simulink library "RF_transformations"  (R2020b)
settings: Solver=VariableStepAuto  StartTime=0.0  StopTime=10.0  RelTol=1e-3
settings Model: Creator=matteolarcher  LastModifiedBy=matteolarcher

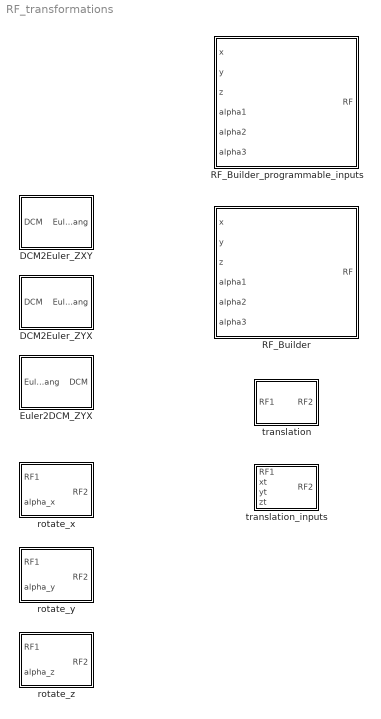
== system RF_transformations ==
  DCM2Euler_ZXY : MATLAB Function  TreatAsAtomicUnit=on
  DCM2Euler_ZYX : MATLAB Function  TreatAsAtomicUnit=on
  Euler2DCM_ZYX : MATLAB Function  TreatAsAtomicUnit=on
  RF_Builder : MATLAB Function  TreatAsAtomicUnit=on  mask{order_selector=['Z','Y','X']}
      mask prompts: order_selector "Rotation order"
      mask init:
      | switch order_selector
      |     case 1
      |         order = [1,2,3];
      |     case 2
      |         order = [1,3,2];
      |     case 3
      |         order = [2,1,3];
      |     case 4
      |         order = [2,3,1];
      |     case 5
      |         order = [3,2,1];
      |     case 6
      |         order = [3,1,2];
      |     case 7
      |         order = [1,2,1];
      |     case 8
      |         order = [1,3,1];
      |     case 9
      |         order = [2,1,2];
      |     case 10
      |         order = [2,3,2];
      |     case 11
      |         order = [3,1,3];
      |     case 12
      |         order = [3,2,3];
      | end
  RF_Builder_programmable_inputs : MATLAB Function  TreatAsAtomicUnit=on  mask{order_input=[3,2,1]}
      mask prompts: order_input "Rotation order"
      mask init:
      | % check input
      | if sum(order_input==1) ~= 1 || sum(order_input==2) ~= 1 || sum(order_input==3) ~= 1
      |     error("input must be provided in the format: [<axis1>,<axis2>,<axis3>], where axis can be 1 for X axis, 2 for Y axis or 3 fro Z axis");
      | end
      | 
      | order = order_input; 
      | 
      | % % assign rotation order
      | % order = [(1*(order_input(1)=='X'))+(2*(order_input(1)=='Y'))+(3*(order_input(1)=='Z')),...
      | %          (1*(order_input(2)=='X'))+(2*(order_input(2)=='Y'))+(3*(order_input(2)=='Z')),...
      | %          (1*(order_input(3)=='X'))+(2*(order_input(3)=='Y'))+(3*(order_input(3)=='Z'))];
  rotate_x : MATLAB Function  TreatAsAtomicUnit=on
  rotate_y : MATLAB Function  TreatAsAtomicUnit=on
  rotate_z : MATLAB Function  TreatAsAtomicUnit=on
  translation : MATLAB Function  TreatAsAtomicUnit=on  mask{xt=0, yt=0, zt=0}
      mask prompts: xt "x"; yt "y"; zt "z"
  translation_inputs : MATLAB Function  TreatAsAtomicUnit=on

== matlab function RF_transformations/DCM2Euler_ZYX ==
  data: DCM input; Euler_ang output
function Euler_ang  = fcn(DCM)

alpha_z = atan2(DCM(2,1),DCM(1,1));
alpha_y = -asin(DCM(3,1));
alpha_x = atan2(DCM(3,2),DCM(3,3));

Euler_ang = [alpha_z,alpha_y,alpha_x];

== matlab function RF_transformations/Euler2DCM_ZYX ==
  data: Euler_ang input; DCM output
function DCM  = fcn(Euler_ang)

alpha_z = Euler_ang(1);
alpha_y = Euler_ang(2);
alpha_x = Euler_ang(3);

DCM = [cos(alpha_z) * cos(alpha_y) -sin(alpha_z) * cos(alpha_x) + cos(alpha_z) * sin(alpha_y) * sin(alpha_x) sin(alpha_z) * sin(alpha_x) + cos(alpha_z) * sin(alpha_y) * cos(alpha_x); sin(alpha_z) * cos(alpha_y) cos(alpha_z) * cos(alpha_x) + sin(alpha_z) * sin(alpha_y) * sin(alpha_x) -cos(alpha_z) * sin(alpha_x) + sin(alpha_z) * sin(alpha_y) * cos(alpha_x); -sin(alpha_y) cos(alpha_y) * sin(alpha_x) cos(alpha_y) * cos(alpha_x)];

== matlab function RF_transformations/DCM2Euler_ZXY ==
  data: DCM input; Euler_ang output
function Euler_ang  = fcn(DCM)

alpha_x = asin(DCM(3,2));
alpha_y = -atan2(DCM(3,1),DCM(3,3));
alpha_z = -atan2(DCM(1,2),DCM(2,2));

Euler_ang = [alpha_z,alpha_x,alpha_y];

== matlab function RF_transformations/RF_Builder ==
  data: x input; RF output size=[4,4]; y input; z input; alpha1 input; alpha2 input; alpha3 input; order parameter
function RF = RF_Builder(x,y,z,alpha1,alpha2,alpha3,order)

RF = [1 0 0 x; 0 1 0 y; 0 0 1 z; 0 0 0 1;];

thetas = [alpha1,alpha2,alpha3];

for i = 1:3
    
    switch order(i)
        case 1
            theta = thetas(i);
            RX = [1 0 0 0; 0 cos(theta) -sin(theta) 0; 0 sin(theta) cos(theta) 0; 0 0 0 1;];
            RF = RF * RX;
        case 2
            theta = thetas(i);
            RY = [cos(theta) 0 sin(theta) 0; 0 1 0 0; -sin(theta) 0 cos(theta) 0; 0 0 0 1;];
            RF = RF * RY;
        case 3
            theta = thetas(i);
            RZ = [cos(theta) -sin(theta) 0 0; sin(theta) cos(theta) 0 0; 0 0 1 0; 0 0 0 1;];
            RF = RF * RZ;
    end
    
end

== matlab function RF_transformations/RF_Builder_programmable_inputs ==
  data: x input; RF output size=[4,4]; y input; z input; alpha1 input; alpha2 input; alpha3 input; order parameter
function RF = RF_Builder(x,y,z,alpha1,alpha2,alpha3,order)

RF = [1 0 0 x; 0 1 0 y; 0 0 1 z; 0 0 0 1;];

thetas = [alpha1,alpha2,alpha3];

for i = 1:3
    
    switch order(i)
        case 1
            theta = thetas(i);
            RX = [1 0 0 0; 0 cos(theta) -sin(theta) 0; 0 sin(theta) cos(theta) 0; 0 0 0 1;];
            RF = RF * RX;
        case 2
            theta = thetas(i);
            RY = [cos(theta) 0 sin(theta) 0; 0 1 0 0; -sin(theta) 0 cos(theta) 0; 0 0 0 1;];
            RF = RF * RY;
        case 3
            theta = thetas(i);
            RZ = [cos(theta) -sin(theta) 0 0; sin(theta) cos(theta) 0 0; 0 0 1 0; 0 0 0 1;];
            RF = RF * RZ;
    end
    
end

== matlab function RF_transformations/translation_inputs ==
  data: RF1 input size=[4,4]; RF2 output size=[4,4]; xt input; yt input; zt input
function RF2 = translation(RF1,xt, yt, zt)
RF2 = RF1*(eye(4) + [zeros(4,3) [xt,yt,zt,0]']);
end

== matlab function RF_transformations/rotate_y ==
  data: RF1 input size=[4,4]; RF2 output size=[4,4]; alpha_y input
function RF2  = fcn(RF1,alpha_y)



DCM = [cos(alpha_y) 0 -sin(alpha_y) 0; 0 1 0 0; sin(alpha_y) 0 cos(alpha_y) 0; 0 0 0 1];

RF2 = RF1 * DCM;

== matlab function RF_transformations/rotate_x ==
  data: RF1 input size=[4,4]; RF2 output size=[4,4]; alpha_x input
function RF2  = fcn(RF1,alpha_x)



DCM = [1 0 0 0; 0 cos(alpha_x) sin(alpha_x) 0; 0 -sin(alpha_x) cos(alpha_x) 0; 0 0 0 1];

RF2 = RF1 * DCM;

== matlab function RF_transformations/rotate_z ==
  data: RF1 input size=[4,4]; RF2 output size=[4,4]; alpha_z input
function RF2  = fcn(RF1,alpha_z)



DCM = [cos(alpha_z) sin(alpha_z) 0 0; -sin(alpha_z) cos(alpha_z) 0 0; 0 0 1 0; 0 0 0 1];

RF2 = RF1 * DCM;

== matlab function RF_transformations/translation ==
  data: RF1 input size=[4,4]; RF2 output size=[4,4]; xt parameter; yt parameter; zt parameter
function RF2 = translation(RF1,xt, yt, zt)
RF2 = RF1*(eye(4) + [zeros(4,3) [xt,yt,zt,0]']);
end
